simulink model "shejidianji"  (R2024b)
settings: Solver=VariableStepAuto  StartTime=0.0  StopTime=50  RelTol=1e-3
libraries: Solver_SF x1
settings Model: Creator=28677  LastModifiedBy=28677

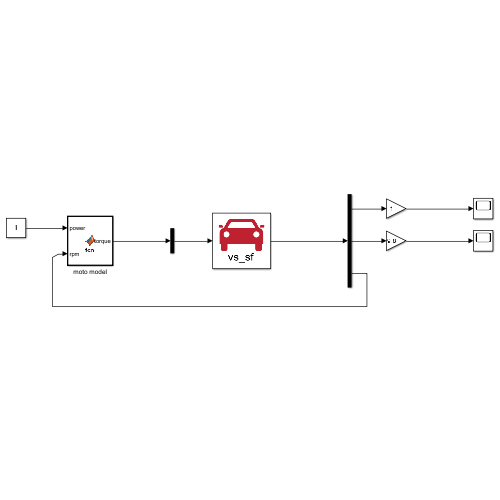
[thumbnail: Simulink's stored preview of the top-level diagram]
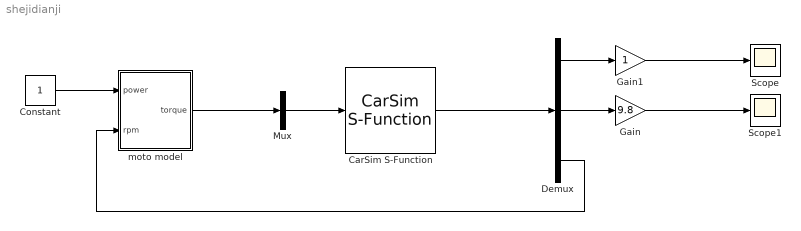
== system shejidianji ==
  CarSim S-Function : Solver_SF/CarSim S-Function  Priority=1  SIMFILE=simfile.sim  Run_RTs=off  vs_state_ind=Run  StopMode_ind=Vehicle Model
  Constant : Constant
  Demux : Demux  Outputs=3
  Gain : Gain  Gain=9.8
  Gain1 : Gain
  Mux : Mux  Inputs=1
  Scope : Scope
  Scope1 : Scope
  moto model : MATLAB Function  TreatAsAtomicUnit=on
  wires:
  Mux/1 -> CarSim S-Function/1
  CarSim S-Function/1 -> Demux/1
  moto model/1(torque) -> Mux/1
  Demux/3 -> moto model/2(rpm)
  Demux/2 -> Gain/1
  Gain1/1 -> Scope/1
  Gain/1 -> Scope1/1
  Demux/1 -> Gain1/1
  Constant/1 -> moto model/1(power)

== matlab function shejidianji/moto model ==
  data: power input; torque output; rpm input
function torque = fcn(power,rpm)
Tmax=380*power;
if(rpm<=4523)
    torque=Tmax;
else
    torque=Tmax*4523/rpm;
end
end
